simulink model "Clarks_invers_Clarks"  (R2020a)
settings: Solver=VariableStepAuto  StartTime=0.0  StopTime=.1  RelTol=1e-3
settings Model: Creator=hp  LastModifiedBy=hp

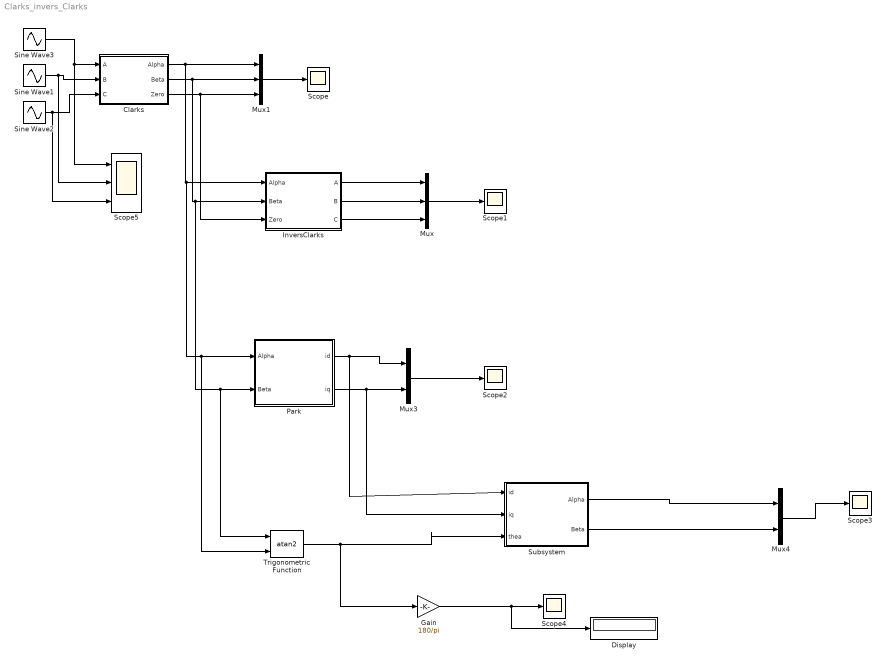
== system Clarks_invers_Clarks ==
  Clarks : Subsystem
  Display : Display
  Gain : Gain  Gain=180/pi
  InversClarks : Subsystem
  Mux : Mux  Inputs=3
  Mux1 : Mux  Inputs=3
  Mux3 : Mux  Inputs=2
  Mux4 : Mux  Inputs=2
  Park : Subsystem
  Scope{,1..4} (5 alike) : Scope
  Scope5 : Scope  NumInputPorts=3
  Sine Wave1 : Sin  Frequency=2*pi*50  Phase=(2*pi)/3  SampleTime=5e-6
  Sine Wave2 : Sin  Frequency=2*pi*50  Phase=(4*pi)/3  SampleTime=5e-6
  Sine Wave3 : Sin  Frequency=2*pi*50  SampleTime=5e-6
  Subsystem : Subsystem
  Trigonometric Function : Trigonometry  Operator=atan2
  wires:
  Mux1/1 -> Scope/1
  Sine Wave3/1 -> Scope5/1, Clarks/1(A)
  Sine Wave1/1 -> Scope5/2, Clarks/2(B)
  Sine Wave2/1 -> Scope5/3, Clarks/3(C)
  Clarks/1(Alpha) -> Trigonometric Function/2, Park/1(Alpha), InversClarks/1(Alpha), Mux1/1
  Clarks/2(Beta) -> Trigonometric Function/1, Park/2(Beta), InversClarks/2(Beta), Mux1/2
  Clarks/3(Zero) -> InversClarks/3(Zero), Mux1/3
  Mux/1 -> Scope1/1
  InversClarks/1(A) -> Mux/1
  InversClarks/2(B) -> Mux/2
  InversClarks/3(C) -> Mux/3
  Mux3/1 -> Scope2/1
  Park/1(id) -> Subsystem/1(id), Mux3/1
  Park/2(iq) -> Subsystem/2(iq), Mux3/2
  Mux4/1 -> Scope3/1
  Subsystem/1(Alpha) -> Mux4/1
  Subsystem/2(Beta) -> Mux4/2
  Trigonometric Function/1 -> Gain/1, Subsystem/3(thea)
  Gain/1 -> Display/1, Scope4/1

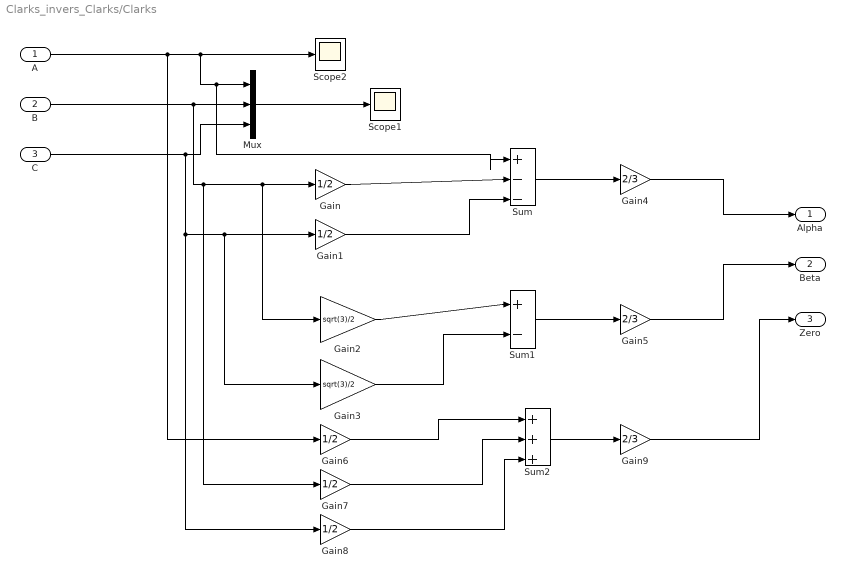
== system Clarks_invers_Clarks/Clarks ==
  A : Inport
  B : Inport  Port=2
  C : Inport  Port=3
  Gain{,1,6..8} (5 alike) : Gain  Gain=1/2
  Gain2 : Gain  Gain=sqrt(3)/2
  Gain3 : Gain  Gain=sqrt(3)/2
  Gain4 : Gain  Gain=2/3
  Gain5 : Gain  Gain=2/3
  Gain9 : Gain  Gain=2/3
  Mux : Mux  Inputs=3
  Scope1 : Scope
  Scope2 : Scope
  Sum : Sum  Inputs=|+--
  Sum1 : Sum  Inputs=|+-
  Sum2 : Sum  Inputs=|+++
  Alpha : Outport
  Beta : Outport  Port=2
  Zero : Outport  Port=3
  wires:
  A/1 -> Gain6/1, Sum/1, Mux/1, Scope2/1
  Gain8/1 -> Sum2/3
  Mux/1 -> Scope1/1
  Gain/1 -> Sum/2
  Gain4/1 -> Alpha/1
  Gain3/1 -> Sum1/2
  B/1 -> Gain7/1, Gain2/1, Gain/1, Mux/2
  C/1 -> Gain8/1, Gain3/1, Gain1/1, Mux/3
  Sum1/1 -> Gain5/1
  Gain7/1 -> Sum2/2
  Gain2/1 -> Sum1/1
  Sum2/1 -> Gain9/1
  Gain6/1 -> Sum2/1
  Sum/1 -> Gain4/1
  Gain1/1 -> Sum/3
  Gain5/1 -> Beta/1
  Gain9/1 -> Zero/1

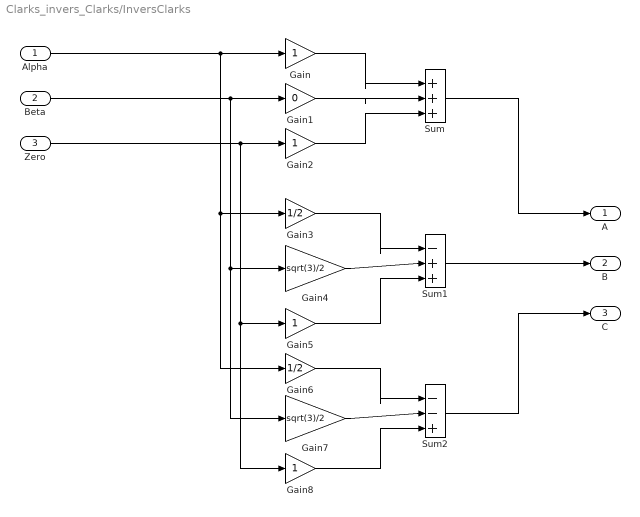
== system Clarks_invers_Clarks/InversClarks ==
  Alpha : Inport
  Beta : Inport  Port=2
  Zero : Inport  Port=3
  Gain{,2,5,8} (4 alike) : Gain
  Gain1 : Gain  Gain=0
  Gain3 : Gain  Gain=1/2
  Gain4 : Gain  Gain=sqrt(3)/2
  Gain6 : Gain  Gain=1/2
  Gain7 : Gain  Gain=sqrt(3)/2
  Sum : Sum  Inputs=|+++
  Sum1 : Sum  Inputs=|-++
  Sum2 : Sum  Inputs=|--+
  A : Outport
  B : Outport  Port=2
  C : Outport  Port=3
  wires:
  Gain5/1 -> Sum1/3
  Gain/1 -> Sum/1
  Gain4/1 -> Sum1/2
  Gain8/1 -> Sum2/3
  Sum/1 -> A/1
  Gain6/1 -> Sum2/1
  Zero/1 -> Gain8/1, Gain5/1, Gain2/1
  Alpha/1 -> Gain6/1, Gain3/1, Gain/1
  Beta/1 -> Gain7/1, Gain4/1, Gain1/1
  Gain1/1 -> Sum/2
  Gain2/1 -> Sum/3
  Gain7/1 -> Sum2/2
  Gain3/1 -> Sum1/1
  Sum2/1 -> C/1
  Sum1/1 -> B/1

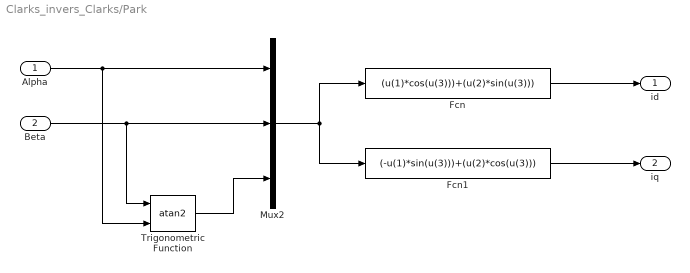
== system Clarks_invers_Clarks/Park ==
  Alpha : Inport
  Beta : Inport  Port=2
  Fcn : Fcn  Expr=(u(1)*cos(u(3)))+(u(2)*sin(u(3)))
  Fcn1 : Fcn  Expr=(-u(1)*sin(u(3)))+(u(2)*cos(u(3)))
  Mux2 : Mux  Inputs=3
  Trigonometric Function : Trigonometry  Operator=atan2
  id : Outport
  iq : Outport  Port=2
  wires:
  Beta/1 -> Mux2/2, Trigonometric Function/1
  Alpha/1 -> Mux2/1, Trigonometric Function/2
  Fcn1/1 -> iq/1
  Mux2/1 -> Fcn1/1, Fcn/1
  Trigonometric Function/1 -> Mux2/3
  Fcn/1 -> id/1

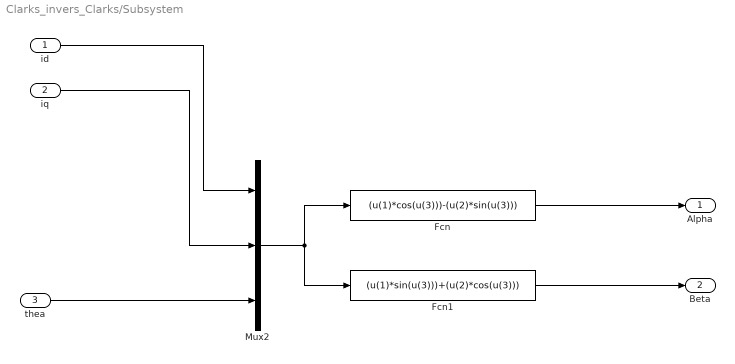
== system Clarks_invers_Clarks/Subsystem ==
  id : Inport
  iq : Inport  Port=2
  thea : Inport  Port=3
  Fcn : Fcn  Expr=(u(1)*cos(u(3)))-(u(2)*sin(u(3)))
  Fcn1 : Fcn  Expr=(u(1)*sin(u(3)))+(u(2)*cos(u(3)))
  Mux2 : Mux  Inputs=3
  Alpha : Outport
  Beta : Outport  Port=2
  wires:
  thea/1 -> Mux2/3
  Mux2/1 -> Fcn1/1, Fcn/1
  id/1 -> Mux2/1
  iq/1 -> Mux2/2
  Fcn1/1 -> Beta/1
  Fcn/1 -> Alpha/1
